simulink model "consensus_leader"  (Simulink 7.8)
settings: Solver=ode45  StartTime=0.0  StopTime=10.0  RelTol=1e-3
settings Model: Creator=chepeadan  LastModifiedBy=Tigervilla
settings DebuggingCC: FcnCallInpInsideContextMsg=Use local settings  StrictBusMsg=Warning

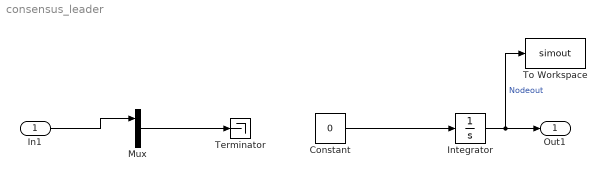
== system consensus_leader ==
  In1 : Inport
  Constant : Constant  Value=0
  Integrator : Integrator  InitialCondition=50*rand()
  Mux : Mux  Inputs=2
  Terminator : Terminator
  To Workspace : ToWorkspace  VariableName=simout  SampleTime=-1  SaveFormat=Structure With Time
  Out1 : Outport
  wires:
  In1/1 -> Mux/1
  Mux/1 -> Terminator/1
  Integrator/1 -> Out1/1, To Workspace/1  "Nodeout"
  Constant/1 -> Integrator/1
